simulink model "dynamics"  (R2022a)
settings: Solver=VariableStepAuto  StartTime=0.0  StopTime=10.0  RelTol=1e-3
values from neighbouring files (symbols this model uses):
  A = [0 0.3 0.4 0.3; 0.3 0 0.5 0; 0.4 0.5 0 0.3; 0.3 0 0.3 0]    [InitialInputsGenerate.m]    (also in initializer.m)
  b = [0.3 0.2 0.5 0.4]    [InitialInputsGenerate.m]    (also in initializer.m)
  c = [9.0 7.0 11.0 7.0]    [InitialInputsGenerate.m]    (also in initializer.m)
  x0 = [16.5 16.5 16.5 16.5]    [InitialInputsGenerate.m]    (also in initializer.m)
settings Model: Creator=Michael  LastModifiedBy=Michael

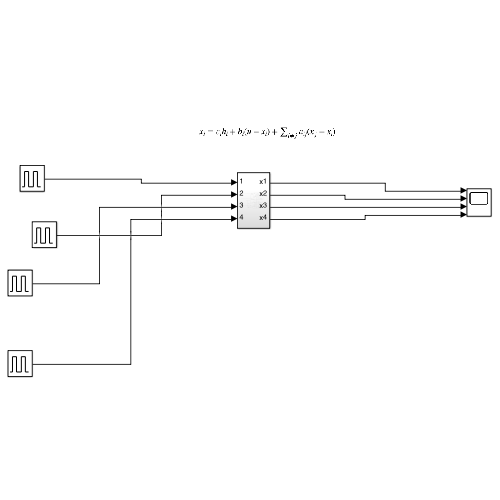
[thumbnail: Simulink's stored preview of the top-level diagram]
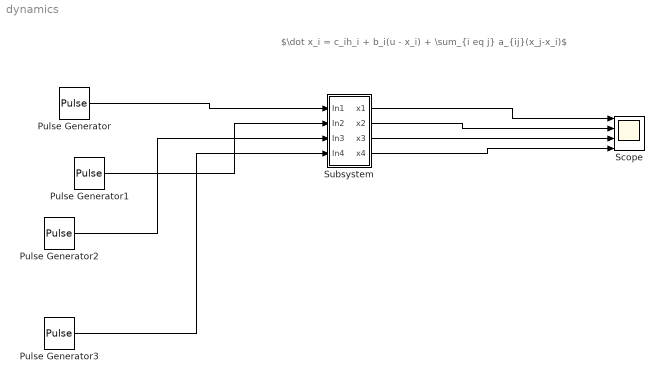
== system dynamics ==
  note: $\dot x_i = c_ih_i + b_i(u - x_i) + \sum_{i\neq j} a_{ij}(x_j-x_i)$
  Pulse Generator : DiscretePulseGenerator  PulseType=Time based  PulseWidth=50
  Pulse Generator1 : DiscretePulseGenerator  PulseType=Time based  PulseWidth=50  PhaseDelay=1
  Pulse Generator2 : DiscretePulseGenerator  PulseType=Time based  PulseWidth=50  PhaseDelay=1
  Pulse Generator3 : DiscretePulseGenerator  PulseType=Time based  PulseWidth=50
  Scope : Scope  NumInputPorts=4
  Subsystem : Subsystem
  wires:
  Pulse Generator/1 -> Subsystem/1(In1)
  Pulse Generator1/1 -> Subsystem/2(In2)
  Pulse Generator2/1 -> Subsystem/3(In3)
  Pulse Generator3/1 -> Subsystem/4(In4)
  Subsystem/1(x1) -> Scope/1
  Subsystem/2(x2) -> Scope/2
  Subsystem/3(x3) -> Scope/3
  Subsystem/4(x4) -> Scope/4

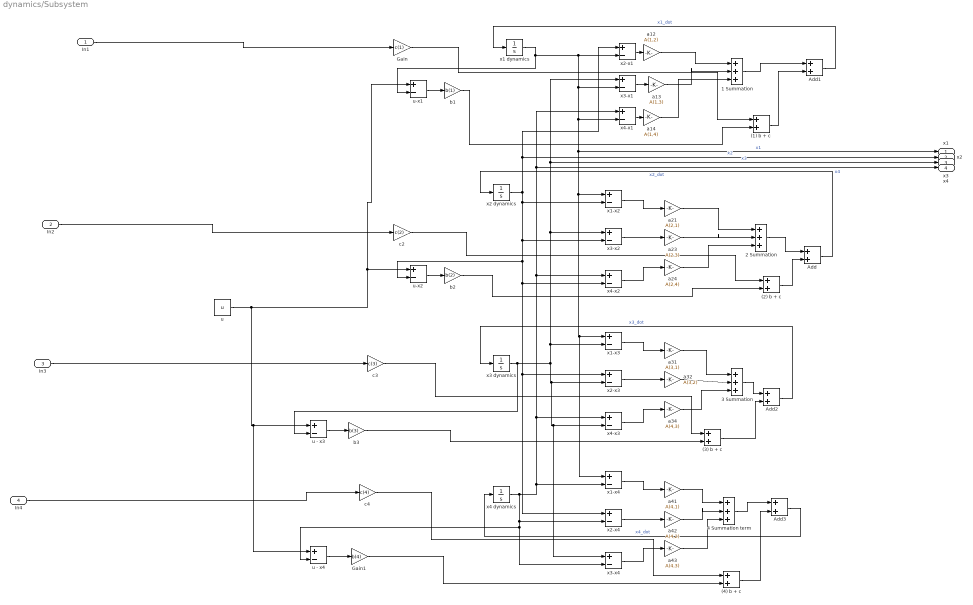
== system dynamics/Subsystem ==
  In1 : Inport
  In2 : Inport  Port=2
  In3 : Inport  Port=3
  In4 : Inport  Port=4
  (1) b + c : Sum
  (2) b + c : Sum
  (3) b + c : Sum
  (4) b + c : Sum
  1 Summation : Sum  Inputs=++|+
  2 Summation : Sum  Inputs=++|+
  3 Summation : Sum  Inputs=++|+
  4 Summation term : Sum  Inputs=++|+
  Add{,1..3} (4 alike) : Sum
  Gain : Gain  Gain=c(1)
  Gain1 : Gain  Gain=b(4)
  a12 : Gain  Gain=A(1,2)
  a13 : Gain  Gain=A(1,3)
  a14 : Gain  Gain=A(1,4)
  a21 : Gain  Gain=A(2,1)
  a23 : Gain  Gain=A(2,3)
  a24 : Gain  Gain=A(2,4)
  a31 : Gain  Gain=A(3,1)
  a32 : Gain  Gain=A(3,2)
  a34 : Gain  Gain=A(4,3)
  a41 : Gain  Gain=A(4,1)
  a42 : Gain  Gain=A(4,2)
  a43 : Gain  Gain=A(4,3)
  b1 : Gain  Gain=b(1)
  b2 : Gain  Gain=b(2)
  b3 : Gain  Gain=b(3)
  c2 : Gain  Gain=c(2)
  c3 : Gain  Gain=c(3)
  c4 : Gain  Gain=c(4)
  u : Constant  Value=u
  u - x3 : Sum  Inputs=+-
  u - x4 : Sum  Inputs=+-
  u-x1 : Sum  Inputs=+-
  u-x2 : Sum  Inputs=+-
  x1 dynamics : Integrator  InitialCondition=x0(1)
  x1-x2 : Sum  Inputs=+-
  x1-x3 : Sum  Inputs=+-
  x1-x4 : Sum  Inputs=+-
  x2 dynamics : Integrator  InitialCondition=x0(2)
  x2-x1 : Sum  Inputs=+-
  x2-x3 : Sum  Inputs=+-
  x2-x4 : Sum  Inputs=+-
  x3 dynamics : Integrator  InitialCondition=x0(3)
  x3-x1 : Sum  Inputs=+-
  x3-x2 : Sum  Inputs=+-
  x3-x4 : Sum  Inputs=+-
  x4 dynamics : Integrator  InitialCondition=x0(4)
  x4-x1 : Sum  Inputs=+-
  x4-x2 : Sum  Inputs=+-
  x4-x3 : Sum  Inputs=+-
  x1 : Outport
  x2 : Outport  Port=2
  x3 : Outport  Port=3
  x4 : Outport  Port=4
  wires:
  In3/1 -> c3/1
  (4) b + c/1 -> Add3/2
  a41/1 -> 4 Summation term/1
  u - x4/1 -> Gain1/1
  a42/1 -> 4 Summation term/2
  b2/1 -> (2) b + c/2
  b3/1 -> (3) b + c/2
  In4/1 -> c4/1
  x2-x4/1 -> a42/1
  (3) b + c/1 -> Add2/2
  a31/1 -> 3 Summation/1
  a34/1 -> 3 Summation/3
  4 Summation term/1 -> Add3/1
  a12/1 -> 1 Summation/1
  u - x3/1 -> b3/1
  u-x2/1 -> b2/1
  x2-x1/1 -> a12/1
  Add/1 -> x2 dynamics/1  "x2_dot"
  a21/1 -> 2 Summation/1
  a32/1 -> 3 Summation/2
  x1-x4/1 -> a41/1
  Add1/1 -> x1 dynamics/1  "x1_dot"
  Add2/1 -> x3 dynamics/1  "x3_dot"
  x3-x1/1 -> a13/1
  In1/1 -> Gain/1
  u-x1/1 -> b1/1
  1 Summation/1 -> Add1/1
  x1-x2/1 -> a21/1
  c2/1 -> (2) b + c/1
  b1/1 -> (1) b + c/2
  a24/1 -> 2 Summation/3
  3 Summation/1 -> Add2/1
  (1) b + c/1 -> Add1/2
  In2/1 -> c2/1
  x1-x3/1 -> a31/1
  x4-x2/1 -> a24/1
  2 Summation/1 -> Add/1
  u/1 -> u - x4/1, u - x3/1, u-x1/1, u-x2/1
  a23/1 -> 2 Summation/2
  a14/1 -> 1 Summation/3
  c4/1 -> (4) b + c/1
  x3-x2/1 -> a23/1
  a43/1 -> 4 Summation term/3
  c3/1 -> (3) b + c/1
  x4 dynamics/1 -> x3-x4/2, u - x4/2, x2-x4/2, x4/1, x4-x1/1, x4-x2/1, x4-x3/1, x1-x4/2  "x4"
  x3-x4/1 -> a43/1
  x4-x1/1 -> a14/1
  x2 dynamics/1 -> x2/1, x2-x1/1, x3-x2/2, x2-x4/1, x2-x3/1, x4-x2/2, u-x2/2, x1-x2/2  "x2"
  x1 dynamics/1 -> u-x1/2, x1/1, x1-x4/1, x1-x3/1, x1-x2/1, x4-x1/2, x3-x1/2, x2-x1/2  "x1"
  x2-x3/1 -> a32/1
  Add3/1 -> x4 dynamics/1  "x4_dot"
  x4-x3/1 -> a34/1
  Gain1/1 -> (4) b + c/2
  (2) b + c/1 -> Add/2
  x3 dynamics/1 -> u - x3/2, x3-x4/1, x4-x3/2, x2-x3/2, x1-x3/2, x3/1, x3-x1/1, x3-x2/1  "x3"
  a13/1 -> 1 Summation/2
  Gain/1 -> (1) b + c/1
